simulink model "sf_data_store_memory"  (Simulink 7.7)
settings: Solver=FixedStepDiscrete  StartTime=0.0  StopTime=10.0  FixedStep=1  RelTol=1e-3
settings Model: Creator=schumann  LastModifiedBy=hnine
settings OptimizationCC: InitFltsAndDblsToZero=on
settings DebuggingCC: SaveWithParameterizedLinksMsg=none  SignalResolutionControl=TryResolveAllWithWarning  StrictBusMsg=Warning
settings SFSimCC: SimParseCustomCode=off
settings GRTTargetCC: TargetFcnLib=ansi_tfl_tmw.mat

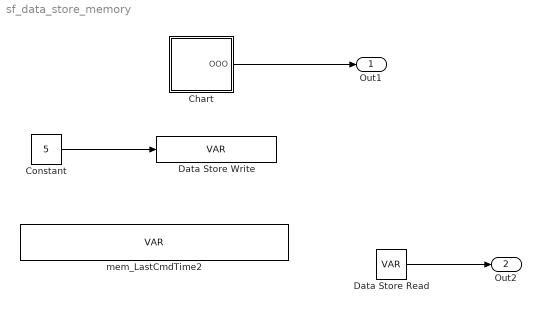
== system sf_data_store_memory ==
  Chart : Stateflow chart  Priority=2  TreatAsAtomicUnit=on
  Constant : Constant  Value=5
  Data Store Read : DataStoreRead  Priority=3  DataStoreName=VAR  SampleTime=0
  Data Store Write : DataStoreWrite  Priority=1  DataStoreName=VAR  SampleTime=1
  mem_LastCmdTime2 : DataStoreMemory  DataStoreName=VAR  ReadBeforeWriteMsg=warning  WriteAfterWriteMsg=warning  WriteAfterReadMsg=warning  OutDataTypeStr=double
  Out1 : Outport  OutDataTypeStr=double
  Out2 : Outport  Port=2
  wires:
  Constant/1 -> Data Store Write/1
  Chart/1(OOO) -> Out1/1
  Data Store Read/1 -> Out2/1

== stateflow chart Chart ==
  state OOO0/
    during: OOO=0;value=value + 1;
  state OOO1/
    OOO=1;
  (default) -> OOO0 : /value = 0;
  OOO0 -> OOO1 : [value>VAR]
  data: value local double; OOO output double; VAR data_store_memory double
